simulink model "weekp1"  (R2021a)
settings: Solver=VariableStepAuto  StartTime=0.0  StopTime=10.0  RelTol=1e-3
values from neighbouring files (symbols this model uses):
  b = 50    [math.m]
  k1 = 50    [math.m]
  k12 = 25    [math.m]
  M1 = 100    [math.m]
  M2 = 50    [math.m]
settings Model: Creator=Nida  LastModifiedBy=Nida

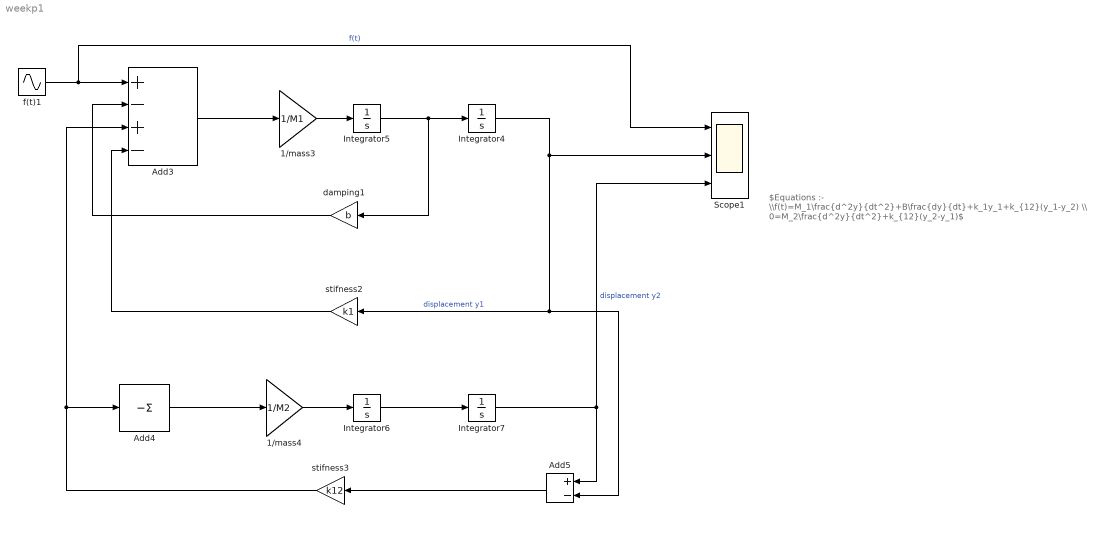
== system weekp1 ==
  note: $Equations :- \\f(t)=M_1\frac{d^2y}{dt^2}+B\frac{dy}{dt}+k_1y_1+k_{12}(y_1-y_2) \\ 0=M_2\frac{d^2y}{dt^2}+k_{12}(y_2-y_1)$
  1/mass3 : Gain  Gain=1/M1
  1/mass4 : Gain  Gain=1/M2
  Add3 : Sum  Inputs=+-+-
  Add4 : Sum  Inputs=-
  Add5 : Sum  Inputs=+-
  Integrator{4..7} (4 alike) : Integrator
  Scope1 : Scope  NumInputPorts=3
  damping1 : Gain  Gain=b
  f(t)1 : Sin  Amplitude=2  Frequency=10  SampleTime=0
  stifness2 : Gain  Gain=k1
  stifness3 : Gain  Gain=k12
  wires:
  damping1/1 -> Add3/2
  stifness2/1 -> Add3/4
  stifness3/1 -> Add3/3, Add4/1
  Integrator7/1 -> Scope1/3, Add5/1  "displacement y2"
  Add4/1 -> 1/mass4/1
  Integrator4/1 -> stifness2/1, Add5/2, Scope1/2  "displacement y1"
  1/mass4/1 -> Integrator6/1
  Integrator6/1 -> Integrator7/1
  Add5/1 -> stifness3/1
  Add3/1 -> 1/mass3/1
  1/mass3/1 -> Integrator5/1
  Integrator5/1 -> Integrator4/1, damping1/1
  f(t)1/1 -> Add3/1, Scope1/1  "f(t)"
